simulink model "classification"  (R2018b)
settings: Solver=VariableStepAuto  StartTime=0.0  StopTime=0.5  MaxStep=0.2  RelTol=1e-4
libraries: powerlib x7, powerlib_meascontrol x4
settings Model: Creator=Edagotti Pavankumar  LastModifiedBy=Edagotti Pavankumar
settings SFSimCC: SimUseLocalCustomCode=off
settings RTWCC: RTWUseLocalCustomCode=off
settings CodeAppCC: StateflowObjectComments=on

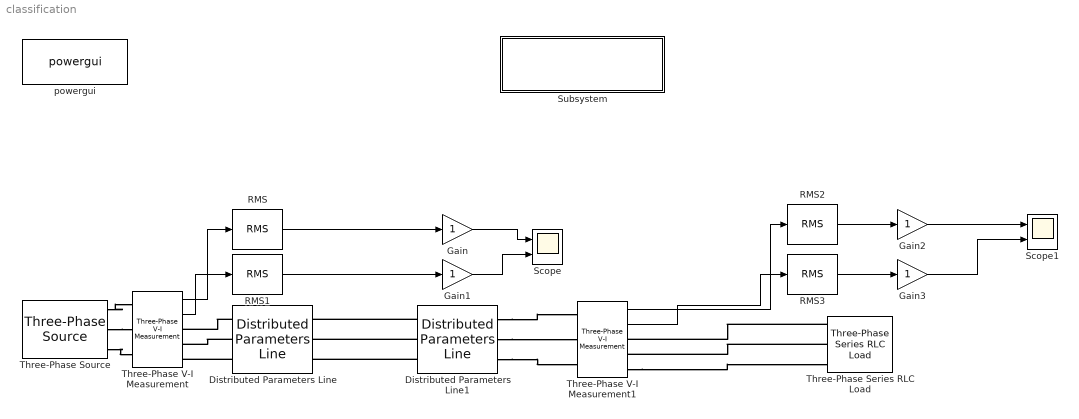
== system classification ==
  Distributed Parameters Line : powerlib/Elements/Distributed Parameters Line  Phases=3  Frequency=50  Resistance=[0.0238 0.3885]  Inductance="[0.0009509508  0.0032508989]"  Capacitance=[12.74e-9 7.751e-9]  Length=20  x1=[1.28621974215375e-12 12009.3478706898 12009.3478706898;314.159265358979 314.159265358979 314.159265358979;-2.38773440156133 0.500551789772784 -1.07024453702211]  x2=[5.55089882970319e-12 12056.765780003 12056.765780003;314.159265358979 314.159265358979 314.159265358979;-2.21306220255309 0.495073809956523 -1.07572251683837]  x3=[4.15158432519257e-13 34.7888853326051 34.7888853326047;314.159265358979 314.159265358979 314.159265358979;2.33217323413566 0.232789483204581 -1.33800684359031]  x4=[4.09969497978707e-13 55.004384786973 55.0043847869731;314.159265358979 314.159265358979 314.159265358979;-0.328772219186676 0.646519807853069 -0.924276518941825]  x5=0.000100394655981083  V1=[1.286e-12 1.201e+04 1.201e+04;314.2 314.2 314.2;-2.388 0.5006 -1.07]  V2=[5.551e-12 1.206e+04 1.206e+04;314.2 314.2 314.2;-2.213 0.4951 -1.076]  I1=[4.152e-13 34.79 34.79;314.2 314.2 314.2;2.332 0.2328 -1.338]  I2=[4.1e-13 55 55;314.2 314.2 314.2;-0.3288 0.6465 -0.9243]  nHarmo=1  Measurements=None
      settings: SourceProductName=Simscape Power Systems
  Distributed Parameters Line1 : powerlib/Elements/Distributed Parameters Line  Phases=3  Frequency=50  Resistance=[0.0238 0.3885]  Inductance="[0.0009509508  0.0032508989]"  Capacitance=[12.74e-9 7.751e-9]  Length=180  x1=[5.55089882970319e-12 12056.765780003 12056.765780003;314.159265358979 314.159265358979 314.159265358979;-2.46538149350497 0.320115895397789 -1.25068043139711]  x2=[5.69796797487546e-12 12237.3789363488 12237.3789363488;314.159265358979 314.159265358979 314.159265358979;2.3583867295888 0.273723793931077 -1.29707253286382]  x3=[6.17217514069241e-14 34.3861016014745 34.3861016014745;314.159265358979 314.159265358979 314.159265358979;-0.0918111850801303 0.0781067687690364 -1.49268955802586]  x4=[3.2153150334582e-14 54.3025641084531 54.3025641084531;314.159265358979 314.159265358979 314.159265358979;2.7528565125387 0.273723793931076 -1.29707253286382]  x5=0.000903551903829747  V1=[5.551e-12 1.206e+04 1.206e+04;314.2 314.2 314.2;-2.465 0.3201 -1.251]  V2=[5.698e-12 1.224e+04 1.224e+04;314.2 314.2 314.2;2.358 0.2737 -1.297]  I1=[6.172e-14 34.39 34.39;314.2 314.2 314.2;-0.09181 0.07811 -1.493]  I2=[3.215e-14 54.3 54.3;314.2 314.2 314.2;2.753 0.2737 -1.297]  nHarmo=1  Measurements=None
      settings: SourceProductName=Simscape Power Systems
  Gain{,1..3} (4 alike) : Gain
  RMS{,1..3} (4 alike) : powerlib_meascontrol/Measurements/RMS  TrueRMS=off  Freq=50  RMSInit=0  Ts=0
  Scope : Scope  NumInputPorts=2
  Scope1 : Scope  NumInputPorts=2
  Subsystem : Subsystem
      settings: OpenFcn=open_system('power_new_palette')
      mask Display: disp(sprintf('Open Simscape Electrical\nSpecialized Power Systems\nPalette Library'));
  Three-Phase Series RLC Load : powerlib/Elements/Three-Phase Series RLC Load  LConnTagsString=A|B|C  Configuration=Y (grounded)  NominalVoltage=11000  Vabc=[1e3 1e3 1e3]  Vabcp=[1e3 1e3 1e3]  NominalFrequency=50  UnbalancedPower=off  ActivePower=100000  InductivePower=0  CapacitivePower=0  Pabc=[10e3 9e3 11e3]  QLabc=[100 90 110]  QCabc=[100 90 110]  Pabcp=[10e3 9e3 11e3]  QLabcp=[100 90 110]  QCabcp=[100 90 110]  Measurements=None  LoadType=constant Z
  Three-Phase V-I Measurement : powerlib/Measurements/Three-Phase V-I Measurement  VoltageMeasurement=phase-to-ground  SetLabelV=off  LabelV=Vabc  Vpu=off  VpuLL=off  CurrentMeasurement=yes  SetLabelI=off  LabelI=Iabc  Ipu=off  Pbase=100e6  Vbase=11e3  OutputType=Complex  PhasorSimulation=off  PSBequivalent=0
  Three-Phase V-I Measurement1 : powerlib/Measurements/Three-Phase V-I Measurement  VoltageMeasurement=phase-to-ground  SetLabelV=off  LabelV=Vabc  Vpu=off  VpuLL=off  CurrentMeasurement=yes  SetLabelI=off  LabelI=Iabc  Ipu=off  Pbase=100e6  Vbase=11e3  OutputType=Complex  PhasorSimulation=off  PSBequivalent=0
  Three-Phase Source : powerlib/Electrical Sources/Three-Phase Source  InternalConnection=Yg  VoltagePhases=off  Voltage=12e3  PhaseAngle=0  Voltage_phases=[11e3 11e3 11e3]/sqrt(3)  PhaseAngles_phases=[0 -120 +120]  Frequency=50  NonIdealSource=on  SpecifyImpedance=on  Resistance=0.8929  Inductance=16.58e-3  ShortCircuitLevel=100e6  BaseVoltage=11e3  XRratio=7  BusType=swing  Pref=10e3  Qref=0  Prefabc=[10e3, 10e3, 10e3]  Qrefabc=[0, 0, 0]  Qmin=-inf  Qmax=inf
  powergui : powerlib/powergui  Priority=1  SimulationMode=Continuous  SampleTime=50e-6  frequency=60  Iterations=50  frequencyindice=50  Pbase=100e6  ErrMax=1e-4  UnitsV=kV  UnitsW=MW  buscounter=0  FunctionMessages=off  echomessages=off  EnableUseOfTLC=off  CurrentSourceSwitches=off  DisableSnubberDevices=off  DisableRonSwitches=off  DisableVfSwitches=off  DisplayEquations=off  SolverType=Tustin/Backward Euler (TBE)  Interpol=off  ExternalGateDelay=off  methode=off  Ts=100  x0status=blocks  SPID=on  SwTol=0  HookPort=off  RestoreLinks=warning  ResistiveCurrentMeasurement=off  Frange=[0:2:500]  Ylog=off  Xlog=on  ShowGrid=off  save=off  variable=ZData  structure=0  ZoomFFT=off  StartTime=0.0  cycles=1  DisplayStyle=1  fundamental=60  FreqAxis=off  MaxFrequency=1000  frequencyindicesteady=1  RmsSteady=1  display=off
  wires:
  Three-Phase V-I Measurement/1 -> RMS/1
  Three-Phase V-I Measurement/2 -> RMS1/1
  RMS/1 -> Gain/1
  RMS1/1 -> Gain1/1
  Gain/1 -> Scope/1
  Gain1/1 -> Scope/2
  RMS2/1 -> Gain2/1
  RMS3/1 -> Gain3/1
  Three-Phase V-I Measurement1/1 -> RMS2/1
  Three-Phase V-I Measurement1/2 -> RMS3/1
  Gain2/1 -> Scope1/1
  Gain3/1 -> Scope1/2
  connections:
  Three-Phase Source/RConn2 -- Three-Phase V-I Measurement/LConn2
  Three-Phase Source/RConn1 -- Three-Phase V-I Measurement/LConn1
  Three-Phase Source/RConn3 -- Three-Phase V-I Measurement/LConn3
  Distributed Parameters Line/LConn1 -- Three-Phase V-I Measurement/RConn1
  Distributed Parameters Line/LConn2 -- Three-Phase V-I Measurement/RConn2
  Distributed Parameters Line/LConn3 -- Three-Phase V-I Measurement/RConn3
  Three-Phase Series RLC Load/LConn2 -- Three-Phase V-I Measurement1/RConn2
  Three-Phase Series RLC Load/LConn1 -- Three-Phase V-I Measurement1/RConn1
  Three-Phase V-I Measurement1/RConn3 -- Three-Phase Series RLC Load/LConn3
  Distributed Parameters Line1/LConn1 -- Distributed Parameters Line/RConn1
  Distributed Parameters Line1/LConn2 -- Distributed Parameters Line/RConn2
  Distributed Parameters Line1/LConn3 -- Distributed Parameters Line/RConn3
  Distributed Parameters Line1/RConn3 -- Three-Phase V-I Measurement1/LConn3
  Distributed Parameters Line1/RConn2 -- Three-Phase V-I Measurement1/LConn2
  Distributed Parameters Line1/RConn1 -- Three-Phase V-I Measurement1/LConn1

== system classification/Subsystem ==
